simulink model "Simulation_Autopilot"  (R2017a)
settings: Solver=VariableStepAuto  StartTime=0.0  StopTime=150  RelTol=1e-3  EnableMultiTasking=on
InitFcn:
  | clear all;
  | load('Parameters.mat');
values from neighbouring files (symbols this model uses):
  altitude = 1750    [Parameters.mat]
  int_time = 10    [Parameters.mat]
  RW_Alt = 0    [Parameters.mat]
  trim_state_hi = [0 0 1750 0 0.149620235853 0 310 0.149620235853 0 0 0 0]    [Parameters.mat]
  velocity = 310    [Parameters.mat]
libraries: simulink x2, aerolibfltsims x1
settings Model: Creator=Y Nie  LastModifiedBy=aelabuser
settings DataIOCC: SaveFormat=Array  SaveOutput=off  SignalLogging=off  DSMLogging=off  TimeSaveName=SimTime
settings OptimizationCC: ExpressionDepthLimit=2147483647  LifeSpan=inf
settings DebuggingCC: UnderspecifiedInitializationDetection=Classic  MergeDetectMultiDrivingBlocksExec=none  FcnCallInpInsideContextMsg=warning  StateNameClashWarn=warning  SFUnexpectedBacktrackingDiag=warning  SFNoUnconditionalDefaultTransitionDiag=warning  SFExecutionAtInitializationDiag=none
settings HardwareCC: ProdBitPerPointer=32  ProdBitPerSizeT=32  ProdBitPerPtrDiffT=32  ProdLargestAtomicFloat=None  ProdIntDivRoundTo=Undefined  ProdEndianess=Unspecified  ProdWordSize=32  ProdHWDeviceType=32-bit Generic
settings ModelReferenceCC: PropagateSignalLabelsOutOfModel=off
settings GRTTargetCC: TargetLangStandard=C89/C90 (ANSI)  GeneratePreprocessorConditionals=Disable all  CombineOutputUpdateFcns=off  GRTInterface=on
settings ConfigComp: CovMetricSettings=dw  CovHtmlReporting=on  CovSaveCumulativeToWorkspaceVar=on  CovSaveSingleToWorkspaceVar=on  CovExternalEMLEnable=off

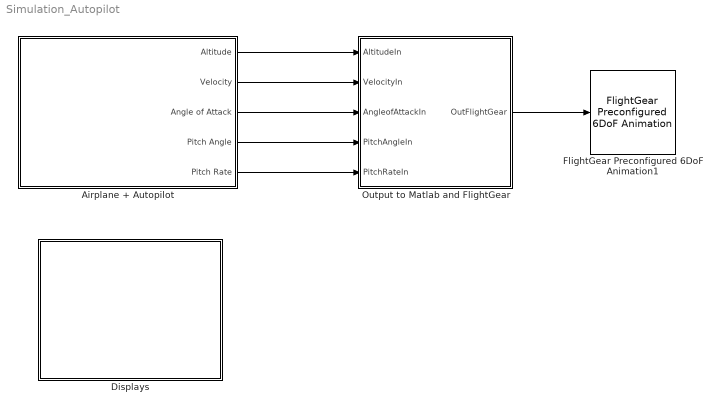
== system Simulation_Autopilot ==
  "Airplane + Autopilot " : Subsystem
      mask Display: image('f16large.JPG');
  Displays : Subsystem
      mask Display: image('f16display.jpg');
  FlightGear Preconfigured 6DoF Animation1 : aerolibfltsims/FlightGear Preconfigured 6DoF Animation  xFlightGearVersion=v2016.3  DestinationIpAddress=146.169.163.108  DestinationPort=5502  SampleTime=0.005
      settings: SourceProductName=Aerospace Blockset
  Output to Matlab and FlightGear : Subsystem
  wires:
  "Airplane + Autopilot "/1(Altitude) -> Output to Matlab and FlightGear/1(AltitudeIn)
  "Airplane + Autopilot "/2(Velocity) -> Output to Matlab and FlightGear/2(VelocityIn)
  "Airplane + Autopilot "/3(Angle of Attack) -> Output to Matlab and FlightGear/3(AngleofAttackIn)
  "Airplane + Autopilot "/4(Pitch Angle) -> Output to Matlab and FlightGear/4(PitchAngleIn)
  "Airplane + Autopilot "/5(Pitch Rate) -> Output to Matlab and FlightGear/5(PitchRateIn)
  Output to Matlab and FlightGear/1(OutFlightGear) -> FlightGear Preconfigured 6DoF Animation1/1

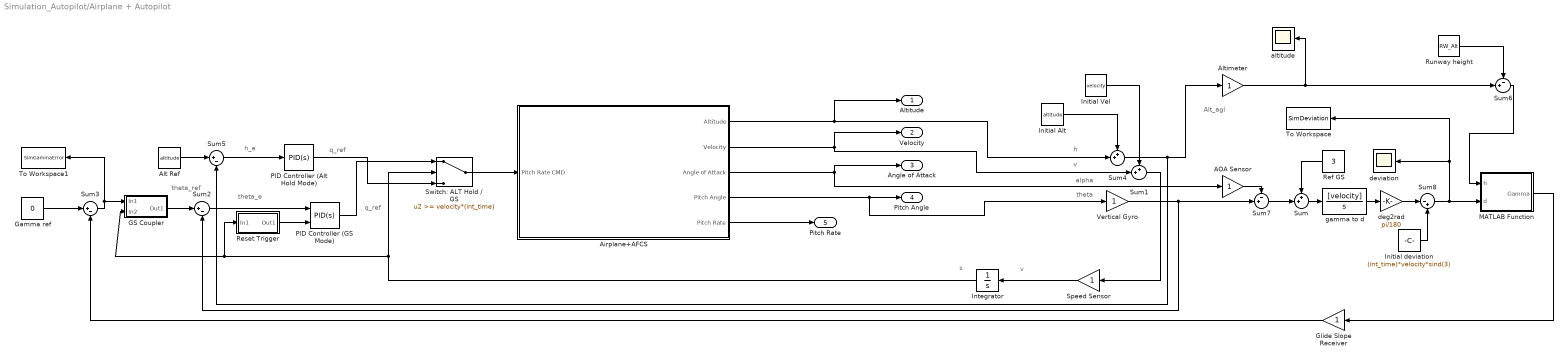
== system Simulation_Autopilot/Airplane + Autopilot  ==
  note: alpha
  note: theta_e
  note: v
  note: q_ref
  note: theta
  note: Alt_agl
  note: theta_ref
  note: h
  note: v
  note: q_ref
  note: s
  note: h_e
  AOA Sensor : Gain
  Airplane+AFCS : Subsystem
      mask Display: image('f163dmodel.jpg');
  Alt Ref : Constant  Value=altitude
  Altimeter : Gain
  GS Coupler : Subsystem
  Gamma ref : Constant  Value=0
  Glide Slope Receiver : Gain
  Initial Alt : Constant  Value=altitude
  Initial Vel : Constant  Value=velocity
  Initial deviation : Constant  Value=(int_time)*velocity*sind(3)
  Integrator : Integrator
  MATLAB Function : MATLAB Function  TreatAsAtomicUnit=on
  PID Controller (Alt Hold Mode) : simulink/Continuous/PID Controller  Controller=PID  TimeDomain=Continuous-time  SampleTime=-1  IntegratorMethod=Forward Euler  FilterMethod=Forward Euler  Form=Parallel  UseFilter=on  ControllerParametersSource=internal  P=0.0003  I=0  D=0.05  N=30  InitialConditionSource=internal  InitialConditionForIntegrator=0  InitialConditionForFilter=0  ExternalReset=none  LimitOutput=off  UpperSaturationLimit=inf  LowerSaturationLimit=-inf  LinearizeAsGain=off  AntiWindupMode=none  Kb=1  TrackingMode=off  Kt=1  PParamMin=[]  PParamMax=[]  IParamMin=[]  IParamMax=[]  DParamMin=[]  DParamMax=[]  NParamMin=[]  NParamMax=[]  KbParamMin=[]  KbParamMax=[]  KtParamMin=[]  KtParamMax=[]  POutMin=[]  POutMax=[]  IOutMin=[]  IOutMax=[]  DOutMin=[]  DOutMax=[]  NOutMin=[]  NOutMax=[]  KbOutMin=[]  KbOutMax=[]  KtOutMin=[]  KtOutMax=[]  IntegratorOutMin=[]  IntegratorOutMax=[]  FilterOutMin=[]  FilterOutMax=[]  SumOutMin=[]  SumOutMax=[]  SumI1OutMin=[]  SumI1OutMax=[]  SumI2OutMin=[]  SumI2OutMax=[]  SumI3OutMin=[]  SumI3OutMax=[]  SumDOutMin=[]  SumDOutMax=[]  SaturationOutMin=[]  SaturationOutMax=[]  IntegratorContinuousStateAttributes=''  IntegratorStateMustResolveToSignalObject=off  IntegratorRTWStateStorageClass=Auto  FilterContinuousStateAttributes=''  FilterStateMustResolveToSignalObject=off  FilterRTWStateStorageClass=Auto  DifferentiatorICPrevScaledInput=0  DifferentiatorOutMin=[]  DifferentiatorOutMax=[]  InitialConditionSetting=State (most efficient)
  PID Controller (GS Mode) : simulink/Continuous/PID Controller  Controller=PID  TimeDomain=Continuous-time  SampleTime=-1  IntegratorMethod=Forward Euler  FilterMethod=Forward Euler  Form=Parallel  UseFilter=on  ControllerParametersSource=internal  P=0.05  I=0.1  D=2  N=160  InitialConditionSource=internal  InitialConditionForIntegrator=0  InitialConditionForFilter=0  ExternalReset=rising  LimitOutput=off  UpperSaturationLimit=inf  LowerSaturationLimit=-inf  LinearizeAsGain=off  AntiWindupMode=none  Kb=1  TrackingMode=off  Kt=1  PParamMin=[]  PParamMax=[]  IParamMin=[]  IParamMax=[]  DParamMin=[]  DParamMax=[]  NParamMin=[]  NParamMax=[]  KbParamMin=[]  KbParamMax=[]  KtParamMin=[]  KtParamMax=[]  POutMin=[]  POutMax=[]  IOutMin=[]  IOutMax=[]  DOutMin=[]  DOutMax=[]  NOutMin=[]  NOutMax=[]  KbOutMin=[]  KbOutMax=[]  KtOutMin=[]  KtOutMax=[]  IntegratorOutMin=[]  IntegratorOutMax=[]  FilterOutMin=[]  FilterOutMax=[]  SumOutMin=[]  SumOutMax=[]  SumI1OutMin=[]  SumI1OutMax=[]  SumI2OutMin=[]  SumI2OutMax=[]  SumI3OutMin=[]  SumI3OutMax=[]  SumDOutMin=[]  SumDOutMax=[]  SaturationOutMin=[]  SaturationOutMax=[]  IntegratorContinuousStateAttributes=''  IntegratorStateMustResolveToSignalObject=off  IntegratorRTWStateStorageClass=Auto  FilterContinuousStateAttributes=''  FilterStateMustResolveToSignalObject=off  FilterRTWStateStorageClass=Auto  DifferentiatorICPrevScaledInput=0  DifferentiatorOutMin=[]  DifferentiatorOutMax=[]  InitialConditionSetting=State (most efficient)
  Ref GS : Constant  Value=3
  Reset Trigger : Subsystem
  Runway height : Constant  Value=RW_Alt
  Speed Sensor : Gain
  Sum : Sum  Inputs=++|
  Sum1 : Sum  Inputs=++|
  Sum2 : Sum  Inputs=|+-
  Sum3 : Sum  Inputs=|+-
  Sum4 : Sum  Inputs=++|
  Sum5 : Sum  Inputs=|+-
  Sum6 : Sum  Inputs=-+|
  Sum7 : Sum  Inputs=-+|
  Sum8 : Sum  Inputs=|-+
  Switch: ALT Hold / GS : Switch  Threshold=velocity*(int_time)
  To Workspace : ToWorkspace  VariableName=SimDeviation  SampleTime=-1
  To Workspace1 : ToWorkspace  VariableName=SimGammaError  SampleTime=-1
  Vertical Gyro : Gain
  altitude : Scope
  deg2rad : Gain  Gain=pi/180
  deviation : Scope
  gamma to d : TransferFcn  Numerator=[velocity]  Denominator=[1 0]
  Altitude : Outport
  Velocity : Outport  Port=2
  Angle of Attack : Outport  Port=3
  Pitch Angle : Outport  Port=4
  Pitch Rate : Outport  Port=5
  wires:
  Airplane+AFCS/5(Pitch Rate) -> Pitch Rate/1
  Sum2/1 -> PID Controller (GS Mode)/1
  deg2rad/1 -> Sum8/1
  Initial deviation/1 -> Sum8/2
  Vertical Gyro/1 -> Sum2/2, Sum7/2
  Sum3/1 -> GS Coupler/1(In1), To Workspace1/1
  Initial Alt/1 -> Sum4/1
  Airplane+AFCS/1(Altitude) -> Sum4/2, Altitude/1
  Ref GS/1 -> Sum/1
  Airplane+AFCS/3(Angle of Attack) -> AOA Sensor/1, Angle of Attack/1
  Sum7/1 -> Sum/2
  Sum/1 -> gamma to d/1
  gamma to d/1 -> deg2rad/1
  Speed Sensor/1 -> Integrator/1
  Sum1/1 -> Speed Sensor/1
  Sum8/1 -> MATLAB Function/2(d), deviation/1, To Workspace/1
  Runway height/1 -> Sum6/1
  Integrator/1 -> GS Coupler/2(In2), Reset Trigger/1(In1), Switch: ALT Hold / GS/2
  Sum4/1 -> Sum5/2, Altimeter/1
  Sum6/1 -> MATLAB Function/1(h)
  Airplane+AFCS/2(Velocity) -> Sum1/2, Velocity/1
  Initial Vel/1 -> Sum1/1
  GS Coupler/1(Out1) -> Sum2/1
  Glide Slope Receiver/1 -> Sum3/2
  Sum5/1 -> PID Controller (Alt Hold Mode)/1
  AOA Sensor/1 -> Sum7/1
  MATLAB Function/1(Gamma) -> Glide Slope Receiver/1
  Altimeter/1 -> altitude/1, Sum6/2
  Airplane+AFCS/4(Pitch Angle) -> Vertical Gyro/1, Pitch Angle/1
  Gamma ref/1 -> Sum3/1
  Reset Trigger/1(Out1) -> PID Controller (GS Mode)/2
  Alt Ref/1 -> Sum5/1
  PID Controller (Alt Hold Mode)/1 -> Switch: ALT Hold / GS/3
  PID Controller (GS Mode)/1 -> Switch: ALT Hold / GS/1
  Switch: ALT Hold / GS/1 -> Airplane+AFCS/1(Pitch Rate CMD)

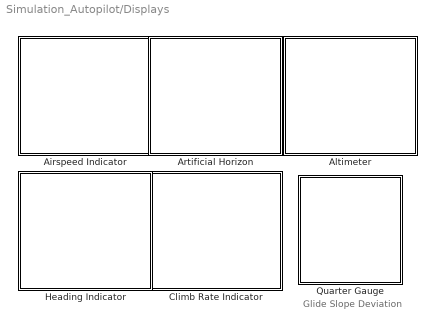
== system Simulation_Autopilot/Displays ==
  note: Glide Slope Deviation
  Airspeed Indicator : Subsystem  DialogController=aeroblksHMICreateDDGDialog  IsWebBlock=on  mask(MWDashboardBlock){webBlockId=b3892bee-502b-44ef-811e-2493f59221ea, webBlockType=airspeedindicator, ShowLibInBrowser=on, ShowInitialText=on, HMISrcModelName=Simulation_Autopilot}
      mask prompts: webBlockId "WebBlock Id"; webBlockType "WebBlock Type"; HMISrcModelName "Source Model"
      mask Help: eval('asbhmihelp(''airspeedindicator'')');
      mask Display:
      | if strcmp(get_param(bdroot(gcb),'BlockDiagramType'), 'library')
      |  image([(matlabroot) '/toolbox/aeroblks/aeroblks/hmi/icons/AirspeedIndicatorIcon.svg'])
      | end
  Altimeter : Subsystem  DialogController=aeroblksHMICreateDDGDialog  IsWebBlock=on  mask(MWDashboardBlock){webBlockId=a0b9298c-5785-4919-b7f8-c7cccb17a8c9, webBlockType=altimeter, ShowLibInBrowser=on, ShowInitialText=on, HMISrcModelName=Simulation_Autopilot}
      mask prompts: webBlockId "WebBlock Id"; webBlockType "WebBlock Type"; HMISrcModelName "Source Model"
      mask Help: eval('asbhmihelp(''altimeter'')');
      mask Display:
      | if strcmp(get_param(bdroot(gcb),'BlockDiagramType'), 'library')
      |  image([(matlabroot) '/toolbox/aeroblks/aeroblks/hmi/icons/AltimeterIcon.svg'])
      | end
  Artificial Horizon : Subsystem  DialogController=aeroblksHMICreateDDGDialog  IsWebBlock=on  mask(MWDashboardBlock){webBlockId=7012071a-1ac7-465e-b6e9-c94febfd6ad2, webBlockType=artificialhorizon, ShowLibInBrowser=on, ShowInitialText=on, HMISrcModelName=Simulation_Autopilot}
      mask prompts: webBlockId "WebBlock Id"; webBlockType "WebBlock Type"; HMISrcModelName "Source Model"
      mask Help: eval('asbhmihelp(''artificialhorizon'')');
      mask Display:
      | if strcmp(get_param(bdroot(gcb),'BlockDiagramType'), 'library')
      |  image([(matlabroot) '/toolbox/aeroblks/aeroblks/hmi/icons/ArtificialHorizonIcon.svg'])
      | end
  Climb Rate Indicator : Subsystem  DialogController=aeroblksHMICreateDDGDialog  IsWebBlock=on  mask(MWDashboardBlock){webBlockId=c36a9585-9208-4b6d-804b-ff501efecac2, webBlockType=climbindicator, ShowLibInBrowser=on, ShowInitialText=on, HMISrcModelName=Simulation_Autopilot}
      mask prompts: webBlockId "WebBlock Id"; webBlockType "WebBlock Type"; HMISrcModelName "Source Model"
      mask Help: eval('asbhmihelp(''climbindicator'')');
      mask Display:
      | if strcmp(get_param(bdroot(gcb),'BlockDiagramType'), 'library')
      |  image([(matlabroot) '/toolbox/aeroblks/aeroblks/hmi/icons/ClimbIndicatorIcon.svg'])
      | end
  Heading Indicator : Subsystem  DialogController=aeroblksHMICreateDDGDialog  IsWebBlock=on  mask(MWDashboardBlock){webBlockId=da6ed19f-560c-41e9-974d-f470a470f1c0, webBlockType=headingindicator, ShowLibInBrowser=on, ShowInitialText=on, HMISrcModelName=Simulation_Autopilot}
      mask prompts: webBlockId "WebBlock Id"; webBlockType "WebBlock Type"; HMISrcModelName "Source Model"
      mask Help: eval('asbhmihelp(''headingindicator'')');
      mask Display:
      | if strcmp(get_param(bdroot(gcb),'BlockDiagramType'), 'library')
      |  image([(matlabroot) '/toolbox/aeroblks/aeroblks/hmi/icons/HeadingIndicatorIcon.svg'])
      | end
  Quarter Gauge : Subsystem  DialogController=hmiCreateDDGDialog  IsWebBlock=on  mask(MWDashboardBlock){webBlockId=35e0a69a-9614-4fa9-a19d-d944fb4c325d, webBlockType=ninetydegreegauge, ShowInLibBrowser=on, ShowInitialText=on, HMISrcModelName=Simulation_Autopilot}
      mask prompts: webBlockId "WebBlock Id"; webBlockType "WebBlock Type"; HMISrcModelName "Source Model"
      mask help: SimulinkHMI:dialogs:NinetydegreeGaugeDialogDesc
      mask Help: helpview([docroot '/mapfiles/simulink.map'], 'hmi_quarter_gauge')
      mask Display:
      | if strcmp(get_param(bdroot(gcb),'BlockDiagramType'), 'library')
      |     image([(matlabroot) '/toolbox/simulink/hmi/icons/NinetyDegreeGauge.png']);
      | end

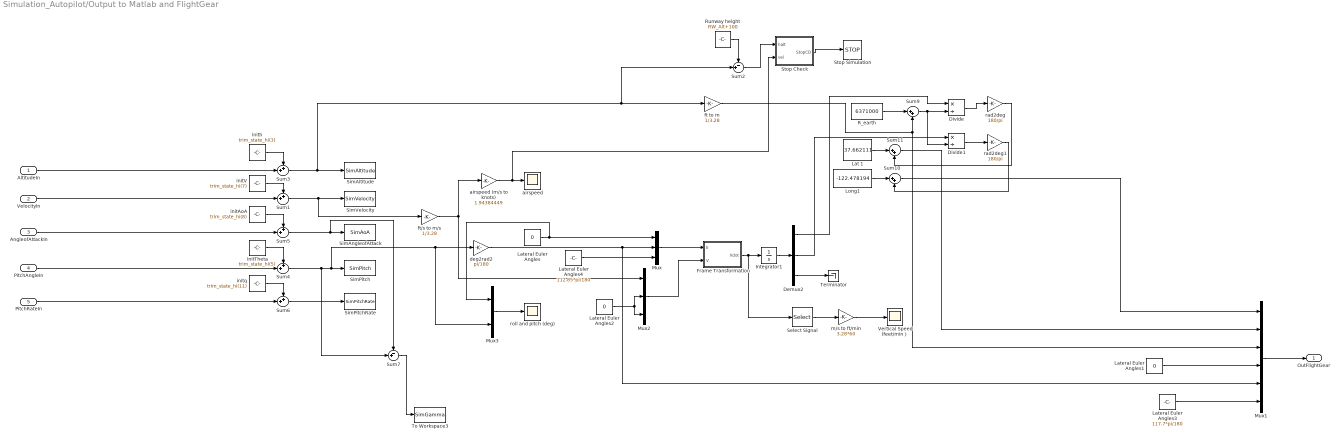
== system Simulation_Autopilot/Output to Matlab and FlightGear ==
  AltitudeIn : Inport
  VelocityIn : Inport  Port=2
  AngleofAttackIn : Inport  Port=3
  PitchAngleIn : Inport  Port=4
  PitchRateIn : Inport  Port=5
  Demux2 : Demux  Outputs=3
  Divide : Product  Inputs=*/
  Divide1 : Product  Inputs=*/
  Frame Transformation : MATLAB Function  TreatAsAtomicUnit=on
  Integrator1 : Integrator
  Lat 1 : Constant  Value=37.662111
  Lateral Euler Angles : Constant  Value=0
  Lateral Euler Angles1 : Constant  Value=0
  Lateral Euler Angles2 : Constant  Value=0
  Lateral Euler Angles3 : Constant  Value=117.7*pi/180
  Lateral Euler Angles4 : Constant  Value=112.85*pi/180
  Long1 : Constant  Value=-122.478194
  Mux : Mux  Inputs=3
  Mux1 : Mux  Inputs=6
  Mux2 : Mux  Inputs=3
  Mux3 : Mux  Inputs=2
  R_earth : Constant  Value=6371000
  Runway height : Constant  Value=RW_Alt+100
  "Select Signal " : Selector  InputPortWidth=3  IndexOptions=Index vector (dialog)  Indices=3  OutputSizes=1
  SimAltitude : ToWorkspace  VariableName=SimAltitude  SampleTime=-1
  SimAngleofAttack : ToWorkspace  VariableName=SimAoA  SampleTime=-1
  SimPitch : ToWorkspace  VariableName=SimPitch  SampleTime=-1
  SimPitchRate : ToWorkspace  VariableName=SimPitchRate  SampleTime=-1
  SimVelocity : ToWorkspace  VariableName=SimVelocity  SampleTime=-1
  Stop Check : MATLAB Function  TreatAsAtomicUnit=on
  Stop Simulation : Stop
  Sum{1,3..6} (5 alike) : Sum  Inputs=++|
  Sum10 : Sum  Inputs=|++
  Sum11 : Sum  Inputs=|++
  Sum2 : Sum  Inputs=-+|
  Sum7 : Sum  Inputs=-+|
  Sum9 : Sum  Inputs=|++
  Terminator : Terminator
  To Workspace3 : ToWorkspace  VariableName=SimGamma  SampleTime=-1
  Vertical Speed (feet/min） : Scope
  "airspeed " : Scope
  airspeed (m/s to knots) : Gain  Gain=1.94384449
  "deg2rad2 " : Gain  Gain=pi/180
  ft to m : Gain  Gain=1/3.28
  ft/s to m/s : Gain  Gain=1/3.28
  initAoA : Constant  Value=trim_state_hi(8)
  initTheta : Constant  Value=trim_state_hi(5)
  initV : Constant  Value=trim_state_hi(7)
  inith : Constant  Value=trim_state_hi(3)
  initq : Constant  Value=trim_state_hi(11)
  "m/s to ft/min " : Gain  Gain=3.28*60
  rad2deg : Gain  Gain=180/pi
  rad2deg1 : Gain  Gain=180/pi
  roll and pitch (deg) : Scope
  OutFlightGear : Outport
  wires:
  inith/1 -> Sum3/1
  Sum6/1 -> SimPitchRate/1
  PitchRateIn/1 -> Sum6/2
  initAoA/1 -> Sum5/1
  PitchAngleIn/1 -> Sum4/2
  Sum1/1 -> SimVelocity/1, ft/s to m/s/1
  initV/1 -> Sum1/1
  initTheta/1 -> Sum4/1
  AltitudeIn/1 -> Sum3/2
  AngleofAttackIn/1 -> Sum5/2
  VelocityIn/1 -> Sum1/2
  initq/1 -> Sum6/1
  Frame Transformation/1(Xdot) -> "Select Signal "/1, Integrator1/1
  Long1/1 -> Sum10/1
  Lateral Euler Angles3/1 -> Mux1/6
  Sum10/1 -> Mux1/1
  Integrator1/1 -> Demux2/1
  Sum9/1 -> Divide1/2, Divide/2
  Demux2/1 -> Divide/1
  ft to m/1 -> Sum9/2, Mux1/3
  Lat 1/1 -> Sum11/1
  Demux2/2 -> Divide1/1
  rad2deg/1 -> Sum11/2
  R_earth/1 -> Sum9/1
  Lateral Euler Angles2/1 -> Mux2/2, Mux2/3
  Lateral Euler Angles1/1 -> Mux1/4
  rad2deg1/1 -> Sum10/2
  Lateral Euler Angles4/1 -> Mux/3
  Lateral Euler Angles/1 -> Mux3/1, Mux/1
  Divide1/1 -> rad2deg1/1
  Mux2/1 -> Frame Transformation/2(V)
  Divide/1 -> rad2deg/1
  Sum3/1 -> Sum2/2, ft to m/1, SimAltitude/1
  Sum11/1 -> Mux1/2
  Mux/1 -> Frame Transformation/1(E)
  "deg2rad2 "/1 -> Mux1/5, Mux/2
  Mux1/1 -> OutFlightGear/1
  Runway height/1 -> Sum2/1
  Sum2/1 -> Stop Check/1(halt)
  ft/s to m/s/1 -> airspeed (m/s to knots)/1, Mux2/1
  airspeed (m/s to knots)/1 -> Stop Check/2(vel), "airspeed "/1
  Mux3/1 -> roll and pitch (deg)/1
  "Select Signal "/1 -> "m/s to ft/min "/1
  "m/s to ft/min "/1 -> Vertical Speed (feet/min）/1
  Sum5/1 -> Sum7/1, SimAngleofAttack/1
  Sum4/1 -> Sum7/2, Mux3/2, "deg2rad2 "/1, SimPitch/1
  Sum7/1 -> To Workspace3/1
  Stop Check/1(StopCD) -> Stop Simulation/1
  Demux2/3 -> Terminator/1

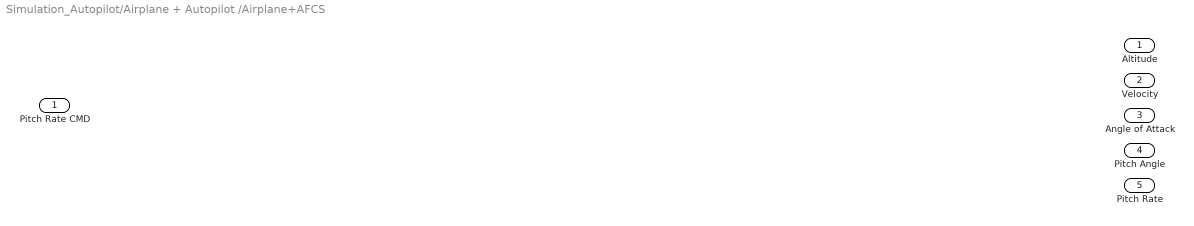
== system Simulation_Autopilot/Airplane + Autopilot /Airplane+AFCS ==
  Pitch Rate CMD : Inport
  Altitude : Outport
  Velocity : Outport  Port=2
  Angle of Attack : Outport  Port=3
  Pitch Angle : Outport  Port=4
  Pitch Rate : Outport  Port=5

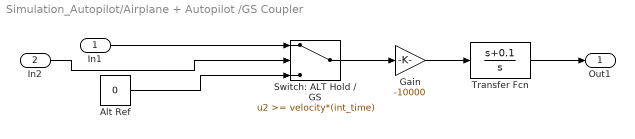
== system Simulation_Autopilot/Airplane + Autopilot /GS Coupler ==
  In1 : Inport
  In2 : Inport  Port=2
  Alt Ref : Constant  Value=0
  Gain : Gain  Gain=-10000
  Switch: ALT Hold / GS : Switch  Threshold=velocity*(int_time)
  Transfer Fcn : TransferFcn  Numerator=[1 0.1]  Denominator=[1 0]
  Out1 : Outport
  wires:
  Gain/1 -> Transfer Fcn/1
  Transfer Fcn/1 -> Out1/1
  Switch: ALT Hold / GS/1 -> Gain/1
  In1/1 -> Switch: ALT Hold / GS/1
  In2/1 -> Switch: ALT Hold / GS/2
  Alt Ref/1 -> Switch: ALT Hold / GS/3

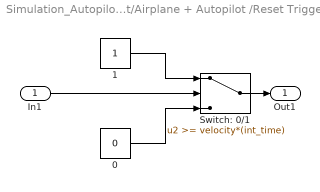
== system Simulation_Autopilot/Airplane + Autopilot /Reset Trigger ==
  In1 : Inport
  0 : Constant  Value=0
  1 : Constant
  Switch: 0/1 : Switch  Threshold=velocity*(int_time)
  Out1 : Outport
  wires:
  0/1 -> Switch: 0/1/3
  Switch: 0/1/1 -> Out1/1
  1/1 -> Switch: 0/1/1
  In1/1 -> Switch: 0/1/2

== system Simulation_Autopilot/Displays/Airspeed Indicator ==

== system Simulation_Autopilot/Displays/Altimeter ==

== system Simulation_Autopilot/Displays/Artificial Horizon ==

== system Simulation_Autopilot/Displays/Climb Rate Indicator ==

== system Simulation_Autopilot/Displays/Heading Indicator ==

== system Simulation_Autopilot/Displays/Quarter Gauge ==

== matlab function Simulation_Autopilot/Output to Matlab and FlightGear/Stop Check ==
  data: halt input; StopCD output; vel input
function StopCD  = StopCheck(halt,vel)
%#codegen
if halt<0 || vel>240
    StopCD=1;
else
    StopCD=0;
end

== matlab function Simulation_Autopilot/Airplane + Autopilot /MATLAB Function ==
  data: h input; Gamma output; d input
function Gamma  = CalcR(h,d)
%#codegen
R=(h)/sind(3)+d/tand(3);
Gamma=(d)/R;

== matlab function Simulation_Autopilot/Output to Matlab and FlightGear/Frame Transformation ==
  data: E input; Xdot output; V input
function Xdot = fcn(E,V)

%#codegen
% transformation from vertical ref. frame to body axes:
Rbv     = [1,  0,         0        ;
           0,  cos(E(1)), sin(E(1));
           0, -sin(E(1)), cos(E(1))]*...
          [cos(E(2)), 0, -sin(E(2));
           0,         1,  0        ;
           sin(E(2)), 0,  cos(E(2))]*...
          [cos(E(3)), sin(E(3)), 0 ;
          -sin(E(3)), cos(E(3)), 0 ;
           0,         0        , 1];


Xdot  = Rbv'*V;

Xdot(3)=-Xdot(3);
